simulink model "z54_dir1"  (R2015a)
settings: Solver=ode45  StartTime=0.0  StopTime=10.0  RelTol=1e-3
settings Model: Creator=Bojana Vasic  LastModifiedBy=Bojana Vasic

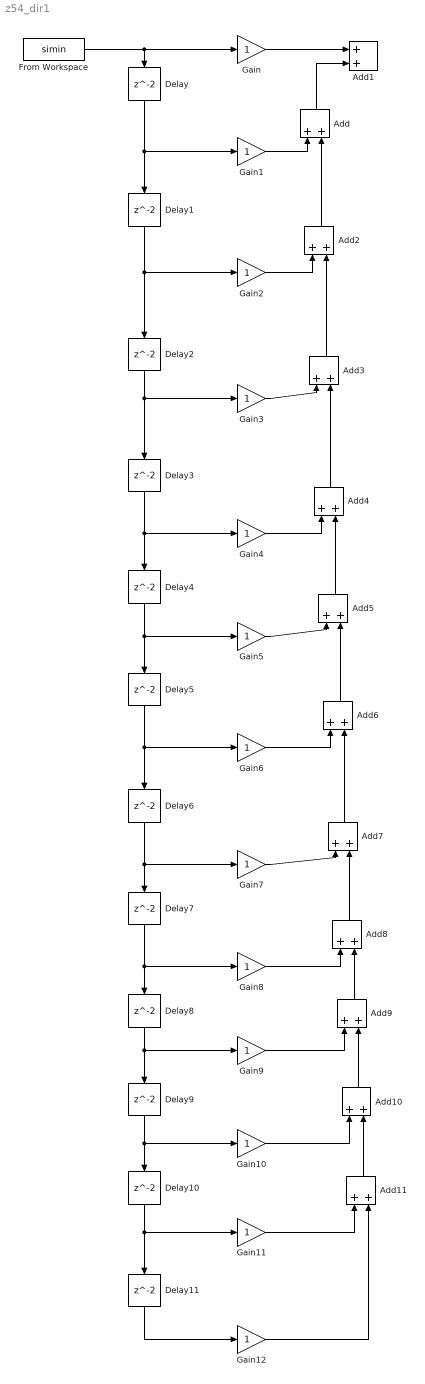
== system z54_dir1 ==
  Add{,1..11} (12 alike) : Sum
  Delay{,1..11} (12 alike) : Delay
  From Workspace : FromWorkspace  VariableName=simin  SampleTime=0
  Gain{,1..12} (13 alike) : Gain
  wires:
  From Workspace/1 -> Delay/1, Gain/1
  Gain/1 -> Add1/1
  Add/1 -> Add1/2
  Gain1/1 -> Add/1
  Delay/1 -> Gain1/1, Delay1/1
  Delay1/1 -> Delay2/1, Gain2/1
  Delay2/1 -> Delay3/1, Gain3/1
  Add2/1 -> Add/2
  Gain2/1 -> Add2/1
  Add3/1 -> Add2/2
  Gain3/1 -> Add3/1
  Delay3/1 -> Delay4/1, Gain4/1
  Gain4/1 -> Add4/1
  Add4/1 -> Add3/2
  Add5/1 -> Add4/2
  Gain5/1 -> Add5/1
  Add6/1 -> Add5/2
  Gain6/1 -> Add6/1
  Add7/1 -> Add6/2
  Delay4/1 -> Delay5/1, Gain5/1
  Delay5/1 -> Delay6/1, Gain6/1
  Delay6/1 -> Gain7/1, Delay7/1
  Gain7/1 -> Add7/1
  Delay7/1 -> Delay8/1, Gain8/1
  Add8/1 -> Add7/2
  Gain8/1 -> Add8/1
  Delay8/1 -> Gain9/1, Delay9/1
  Add9/1 -> Add8/2
  Gain9/1 -> Add9/1
  Delay9/1 -> Delay10/1, Gain10/1
  Delay10/1 -> Delay11/1, Gain11/1
  Gain10/1 -> Add10/1
  Add10/1 -> Add9/2
  Add11/1 -> Add10/2
  Gain11/1 -> Add11/1
  Delay11/1 -> Gain12/1
  Gain12/1 -> Add11/2
